simulink model "SRM_IOT"  (R2024b)
settings: Solver=VariableStepAuto  StartTime=0.0  StopTime=10.0  RelTol=1e-3
undefined symbols (not defined in the file): Ion, Lithium, sigbuilder_block
libraries: spsBreakerLib x120, spsSeriesRLCBranchLib x70, spsBatteryLib x42, spsIdealSwitchLib x33, spsVoltageMeasurementLib x27, slpidlib x17, spsMosfetLib x17, spsPWMGeneratorDCDCLib x11, spsDiodeLib x6, spsCurrentMeasurementLib x4, spsIGBTLib x2, spsThreePhaseSeriesRLCLoadLib x2
(part 4 of 5)

== system SRM_IOT/Grid/Wall charger Connection Box/DC-AC // AC-DC Converter ==
  Controller : Subsystem
  Measurement1 : spsThreePhaseVIMeasurementLib/Three-Phase V-I Measurement  VoltageMeasurement=phase-to-ground  SetLabelV=on  LabelV=Vabc_inv  Vpu=off  VpuLL=off  CurrentMeasurement=yes  SetLabelI=on  LabelI=Iabc_inv  Ipu=off  Pbase=100e6  Vbase=500e3  OutputType=Complex  PhasorSimulation=off  PSBequivalent=0
  PWM Generator (2-Level) : spsPWMGenerator2LevelLib/PWM Generator (2-Level)  ModulatorType=Three-phase bridge (6 pulses)  ModulatorMode=Unsynchronized  Fc=4950  Pc=90  nF=27  MinMax="[ -1  1 ]"  SamplingTechnique=Natural  ModulatingSignals=off  m=0.8  Freq=60  Phase=0  Ts=2.02e-6  ShowCarrierOutport=off
  Parallel Connection control : Constant
  Series RLC Branch2 : spsSeriesRLCBranchLib/Series RLC Branch  LConnTagsString=__new0  RConnTagsString=__new0  BranchType=RC  Resistance=10e3  Inductance=1e-3  SetiL0=off  InitialCurrent=0  Capacitance=1000e-6  Setx0=off  InitialVoltage=0  Measurements=None
  Three-Phase Series RLC Branch : spsThreePhaseSeriesRLCBranchLib/Three-Phase Series RLC Branch  LConnTagsString=A|B|C  RConnTagsString=A|B|C  BranchType=RL  Resistance=0.004332  Inductance=0.0013789184  Capacitance=1e-6  Measurements=None
  Three-Phase Breaker : spsThreePhaseBreakerLib/Three-Phase Breaker  InitialState=open  SwitchA=on  SwitchB=on  SwitchC=on  SwitchTimes="[1/60  5/60]"  External=on  BreakerResistance=0.01  SnubberResistance=1e6  SnubberCapacitance=inf  Measurements=None
  Transformer near home1 : spsThreePhaseSeriesRLCLoadLib/Three-Phase Series RLC Load  LConnTagsString=A|B|C  Configuration=Delta  NominalVoltage=380  Vabc=[1e3 1e3 1e3]  Vabcp=[1e3 1e3 1e3]  NominalFrequency=50  UnbalancedPower=off  ActivePower=100  InductivePower=0  CapacitivePower=5000  Pabc=[10e3 9e3 11e3]  QLabc=[100 90 110]  QCabc=[100 90 110]  Pabcp=[10e3 9e3 11e3]  QLabcp=[100 90 110]  QCabcp=[100 90 110]  Measurements=None  LoadType=constant Z
  Universal Bridge : spsUniversalBridgeLib/Universal Bridge  Arms=3  SnubberResistance=1e5  SnubberCapacitance=inf  Device=IGBT / Diodes  Ron=1e-3  Lon=0  ForwardVoltages="[  0  0  ]"  ForwardVoltage=0  GTOparameters=[ 10e-6 , 20e-6 ]  IGBTparameters=[ 1e-6 , 2e-6 ]  Measurements=None  Measurements_2=None  converterType=Rectifier
  Universal Bridge1 : spsUniversalBridgeLib/Universal Bridge  Arms=3  SnubberResistance=1e5  SnubberCapacitance=inf  Device=Diodes  Ron=1e-3  Lon=0  ForwardVoltages="[  0  0  ]"  ForwardVoltage=0  GTOparameters=[ 10e-6 , 20e-6 ]  IGBTparameters=[ 1e-6 , 2e-6 ]  Measurements=None  Measurements_2=None  converterType=Rectifier
  Discharge_R : PMIOPort  Side=Left
  Discharge_Y : PMIOPort  Port=2  Side=Left
  Discharge_B : PMIOPort  Port=3  Side=Left
  charge_R : PMIOPort  Port=4  Side=Left
  charge_Y : PMIOPort  Port=5  Side=Left
  charge_B : PMIOPort  Port=6  Side=Left
  Discharge + : PMIOPort  Port=7  Side=Right
  Discharge - : PMIOPort  Port=8  Side=Right
  charge+ : PMIOPort  Port=9  Side=Right
  charge- : PMIOPort  Port=10  Side=Right
  wires:
  PWM Generator (2-Level)/1 -> Universal Bridge/1
  Parallel Connection control/1 -> Three-Phase Breaker/1
  [ref] -> PWM Generator (2-Level)/1
  connections:
  Universal Bridge1/LConn2 -- charge_Y/RConn1
  Universal Bridge1/LConn3 -- charge_B/RConn1
  Discharge_Y/RConn1 -- Three-Phase Breaker/RConn2
  Three-Phase Series RLC Branch/RConn1 -- Transformer near home1/LConn1 -- Measurement1/LConn1
  Measurement1/RConn2 -- Three-Phase Breaker/LConn2
  charge-/RConn1 -- Series RLC Branch2/RConn1 -- Universal Bridge1/RConn2
  Three-Phase Series RLC Branch/RConn3 -- Measurement1/LConn3 -- Transformer near home1/LConn3
  Discharge_B/RConn1 -- Three-Phase Breaker/RConn3
  Three-Phase Series RLC Branch/LConn2 -- Universal Bridge/LConn2
  Universal Bridge/LConn1 -- Three-Phase Series RLC Branch/LConn1
  Discharge -/RConn1 -- Universal Bridge/RConn2
  Universal Bridge/LConn3 -- Three-Phase Series RLC Branch/LConn3
  Three-Phase Series RLC Branch/RConn2 -- Measurement1/LConn2 -- Transformer near home1/LConn2
  Discharge +/RConn1 -- Universal Bridge/RConn1
  charge+/RConn1 -- Series RLC Branch2/LConn1 -- Universal Bridge1/RConn1
  Discharge_R/RConn1 -- Three-Phase Breaker/RConn1
  Measurement1/RConn1 -- Three-Phase Breaker/LConn1
  Measurement1/RConn3 -- Three-Phase Breaker/LConn3
  Universal Bridge1/LConn1 -- charge_R/RConn1

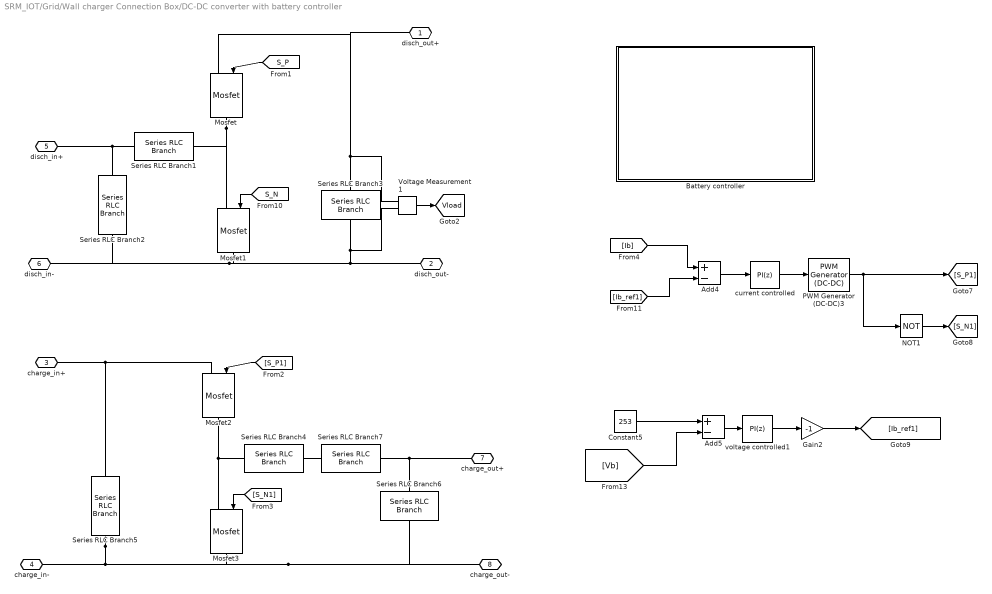
== system SRM_IOT/Grid/Wall charger Connection Box/DC-DC converter with battery controller ==
  Add4 : Sum  Inputs=+-
  Add5 : Sum  Inputs=+-
  Battery controller : Subsystem
  Constant5 : Constant  Value=253
  Gain2 : Gain  Gain=-1
  Mosfet{,1..3} (4 alike) : spsMosfetLib/Mosfet  Ron=0.1  Lon=0  Rd=0.01  Vfd=0  IC=0  Rs=1e5  Cs=inf  Measurements=off
  NOT1 : Logic  Operator=NOT  IconShape=distinctive  AllPortsSameDT=off  OutDataTypeStr=boolean
  PWM Generator (DC-DC)3 : spsPWMGeneratorDCDCLib/PWM Generator (DC-DC)  Fsw=10e3  Ts=5e-6
  Series RLC Branch1 : spsSeriesRLCBranchLib/Series RLC Branch  LConnTagsString=__new0  RConnTagsString=__new0  BranchType=RL  Resistance=1000  Inductance=5.76e-4  SetiL0=off  InitialCurrent=0  Capacitance=1e-6  Setx0=off  InitialVoltage=0  Measurements=None
  Series RLC Branch2 : spsSeriesRLCBranchLib/Series RLC Branch  LConnTagsString=__new0  RConnTagsString=__new0  BranchType=R  Resistance=10  Inductance=1e-3  SetiL0=off  InitialCurrent=0  Capacitance=1000e-6  Setx0=off  InitialVoltage=0  Measurements=None
  Series RLC Branch3 : spsSeriesRLCBranchLib/Series RLC Branch  LConnTagsString=__new0  RConnTagsString=__new0  BranchType=RC  Resistance=0.001  Inductance=1e-3  SetiL0=off  InitialCurrent=0  Capacitance=1000e-6  Setx0=off  InitialVoltage=0  Measurements=None
  Series RLC Branch4 : spsSeriesRLCBranchLib/Series RLC Branch  LConnTagsString=__new0  RConnTagsString=__new0  BranchType=RL  Resistance=0.05  Inductance=5.76e-4  SetiL0=off  InitialCurrent=0  Capacitance=1000e-6  Setx0=off  InitialVoltage=0  Measurements=None
  Series RLC Branch5 : spsSeriesRLCBranchLib/Series RLC Branch  LConnTagsString=__new0  RConnTagsString=__new0  BranchType=RC  Resistance=0.001  Inductance=1e-3  SetiL0=off  InitialCurrent=0  Capacitance=1000e-6  Setx0=off  InitialVoltage=0  Measurements=None
  Series RLC Branch6 : spsSeriesRLCBranchLib/Series RLC Branch  LConnTagsString=__new0  RConnTagsString=__new0  BranchType=RC  Resistance=1e-3  Inductance=1e-3  SetiL0=off  InitialCurrent=0  Capacitance=5600e-6  Setx0=off  InitialVoltage=0  Measurements=None
  Series RLC Branch7 : spsSeriesRLCBranchLib/Series RLC Branch  LConnTagsString=__new0  RConnTagsString=__new0  BranchType=R  Resistance=10  Inductance=1e-3  SetiL0=off  InitialCurrent=0  Capacitance=1000e-6  Setx0=off  InitialVoltage=0  Measurements=None
  Voltage Measurement1 : spsVoltageMeasurementLib/Voltage Measurement  PhasorSimulation=off  OutputType=Complex  PSBequivalent=0
  current controlled : slpidlib/PID Controller  Controller=PI  Form=Parallel  TimeDomain=Discrete-time  UseExternalTs=off  SampleTime=500e-6  IntegratorMethod=Forward Euler  FilterMethod=Forward Euler  ControllerParametersSource=internal  P=0.005  I=10  UseKiTs=off  D=0  UseExternalDerivativeSource=off  N=100  UseFilter=on  TunerSelectOption=Transfer Function Based (PID Tuner App)  InitialConditionSource=internal  InitialConditionForIntegrator=0.54  InitialConditionForFilter=0  DifferentiatorICPrevScaledInput=0  ExternalReset=none  TrackingMode=off  Kt=1  LimitOutput=on  SatLimitsSource=internal  UpperSaturationLimit=0.95  LowerSaturationLimit=0  LinearizeAsGain=on  AntiWindupMode=none  Kb=1  LimitIntegrator=off  UpperIntegratorSaturationLimit=inf  LowerIntegratorSaturationLimit=-inf  POutMin=[]  POutMax=[]  IOutMin=[]  IOutMax=[]  DOutMin=[]  DOutMax=[]  NOutMin=[]  NOutMax=[]  SumOutMin=[]  SumOutMax=[]  SaturationOutMin=[]  SaturationOutMax=[]  PParamMin=[]  PParamMax=[]  IParamMin=[]  IParamMax=[]  DParamMin=[]  DParamMax=[]  NParamMin=[]  NParamMax=[]  KbParamMin=[]  KbParamMax=[]  KtParamMin=[]  KtParamMax=[]  KbOutMin=[]  KbOutMax=[]  KtOutMin=[]  KtOutMax=[]  IntegratorOutMin=[]  IntegratorOutMax=[]  FilterOutMin=[]  FilterOutMax=[]  SumI1OutMin=[]  SumI1OutMax=[]  SumI2OutMin=[]  SumI2OutMax=[]  SumI3OutMin=[]  SumI3OutMax=[]  SumI4OutMin=[]  SumI4OutMax=[]  SumDOutMin=[]  SumDOutMax=[]  DifferentiatorOutMin=[]  DifferentiatorOutMax=[]  FilterDiffOutCoefMin=[]  FilterDiffOutCoefMax=[]  ReciprocalOutMin=[]  ReciprocalOutMax=[]  SumDenOutMin=[]  SumDenOutMax=[]  SumNumOutMin=[]  SumNumOutMax=[]  DivideOutMin=[]  DivideOutMax=[]  UdiffTsProdOutMin=[]  UdiffTsProdOutMax=[]  NTsProdOutMin=[]  NTsProdOutMax=[]  UintegralTsProdOutMin=[]  UintegralTsProdOutMax=[]  UngainTsProdOutMin=[]  UngainTsProdOutMax=[]  ClampingZeroOutDataTypeStr=Inherit: Inherit via back propagation  ClampingZeroOutMin=[]  ClampingZeroOutMax=[]  FilterDenConstantOutDataTypeStr=Inherit: Inherit via back propagation  FilterDenConstantOutMin=[]  FilterDenConstantOutMax=[]  PCopyOutDataTypeStr=Inherit: Inherit via back propagation  PCopyOutMin=[]  PCopyOutMax=[]  NCopyOutDataTypeStr=Inherit: Inherit via back propagation  NCopyOutMin=[]  NCopyOutMax=[]  IntegratorContinuousStateAttributes=''  IntegratorStateMustResolveToSignalObject=off  IntegratorRTWStateStorageClass=Auto  FilterContinuousStateAttributes=''  FilterStateMustResolveToSignalObject=off  FilterRTWStateStorageClass=Auto  ParallelPVariant=InternalParameters  IdealPVariant=Disabled  IVariant=InternalParameters  DVariant=Disabled  IntegratorVariant=Discrete  SatVariant=Enabled  AWVariant=Passthrough  PCopyVariant=Disabled  TRVariant=Disabled  FdbkBlocksVariant=Forward  IdealPFdbkVariant=Disabled  SatFdbkVariant=Disabled  DerivativeFilterVariant=Disabled  NVariant=Disabled  NCopyVariant=Disabled_SignalSpec  FilterICVariant=Disabled  IntegratorICVariant=InternalICs  ExternalResetVariant=Disabled  TRSumVariant=Passthrough  SumFdbkVariant=Disabled  SumVariant=Sum_PI  TsampFilterVariant=InternalTs  TsampNgainVariant=Passthrough  TsampIntegralVariant=Disabled_SignalSpec  ExternalSaturationOutDataTypeStr=Inherit: Same as second input  DerivativeSourceVariant=Disabled  PreIntVariant=InternalPreInt
  voltage controlled1 : slpidlib/PID Controller  Controller=PI  Form=Parallel  TimeDomain=Discrete-time  UseExternalTs=off  SampleTime=500e-6  IntegratorMethod=Forward Euler  FilterMethod=Forward Euler  ControllerParametersSource=internal  P=40  I=2000  UseKiTs=off  D=0  UseExternalDerivativeSource=off  N=100  UseFilter=on  TunerSelectOption=Transfer Function Based (PID Tuner App)  InitialConditionSource=internal  InitialConditionForIntegrator=0  InitialConditionForFilter=0  DifferentiatorICPrevScaledInput=0  ExternalReset=none  TrackingMode=off  Kt=1  LimitOutput=on  SatLimitsSource=internal  UpperSaturationLimit=22  LowerSaturationLimit=0  LinearizeAsGain=on  AntiWindupMode=none  Kb=1  LimitIntegrator=off  UpperIntegratorSaturationLimit=inf  LowerIntegratorSaturationLimit=-inf  POutMin=[]  POutMax=[]  IOutMin=[]  IOutMax=[]  DOutMin=[]  DOutMax=[]  NOutMin=[]  NOutMax=[]  SumOutMin=[]  SumOutMax=[]  SaturationOutMin=[]  SaturationOutMax=[]  PParamMin=[]  PParamMax=[]  IParamMin=[]  IParamMax=[]  DParamMin=[]  DParamMax=[]  NParamMin=[]  NParamMax=[]  KbParamMin=[]  KbParamMax=[]  KtParamMin=[]  KtParamMax=[]  KbOutMin=[]  KbOutMax=[]  KtOutMin=[]  KtOutMax=[]  IntegratorOutMin=[]  IntegratorOutMax=[]  FilterOutMin=[]  FilterOutMax=[]  SumI1OutMin=[]  SumI1OutMax=[]  SumI2OutMin=[]  SumI2OutMax=[]  SumI3OutMin=[]  SumI3OutMax=[]  SumI4OutMin=[]  SumI4OutMax=[]  SumDOutMin=[]  SumDOutMax=[]  DifferentiatorOutMin=[]  DifferentiatorOutMax=[]  FilterDiffOutCoefMin=[]  FilterDiffOutCoefMax=[]  ReciprocalOutMin=[]  ReciprocalOutMax=[]  SumDenOutMin=[]  SumDenOutMax=[]  SumNumOutMin=[]  SumNumOutMax=[]  DivideOutMin=[]  DivideOutMax=[]  UdiffTsProdOutMin=[]  UdiffTsProdOutMax=[]  NTsProdOutMin=[]  NTsProdOutMax=[]  UintegralTsProdOutMin=[]  UintegralTsProdOutMax=[]  UngainTsProdOutMin=[]  UngainTsProdOutMax=[]  ClampingZeroOutDataTypeStr=Inherit: Inherit via back propagation  ClampingZeroOutMin=[]  ClampingZeroOutMax=[]  FilterDenConstantOutDataTypeStr=Inherit: Inherit via back propagation  FilterDenConstantOutMin=[]  FilterDenConstantOutMax=[]  PCopyOutDataTypeStr=Inherit: Inherit via back propagation  PCopyOutMin=[]  PCopyOutMax=[]  NCopyOutDataTypeStr=Inherit: Inherit via back propagation  NCopyOutMin=[]  NCopyOutMax=[]  IntegratorContinuousStateAttributes=''  IntegratorStateMustResolveToSignalObject=off  IntegratorRTWStateStorageClass=Auto  FilterContinuousStateAttributes=''  FilterStateMustResolveToSignalObject=off  FilterRTWStateStorageClass=Auto  ParallelPVariant=InternalParameters  IdealPVariant=Disabled  IVariant=InternalParameters  DVariant=Disabled  IntegratorVariant=Discrete  SatVariant=Enabled  AWVariant=Passthrough  PCopyVariant=Disabled  TRVariant=Disabled  FdbkBlocksVariant=Forward  IdealPFdbkVariant=Disabled  SatFdbkVariant=Disabled  DerivativeFilterVariant=Disabled  NVariant=Disabled  NCopyVariant=Disabled_SignalSpec  FilterICVariant=Disabled  IntegratorICVariant=InternalICs  ExternalResetVariant=Disabled  TRSumVariant=Passthrough  SumFdbkVariant=Disabled  SumVariant=Sum_PI  TsampFilterVariant=InternalTs  TsampNgainVariant=Passthrough  TsampIntegralVariant=Disabled_SignalSpec  ExternalSaturationOutDataTypeStr=Inherit: Same as second input  DerivativeSourceVariant=Disabled  PreIntVariant=InternalPreInt
  disch_out+ : PMIOPort  Side=Left
  disch_out- : PMIOPort  Port=2  Side=Left
  charge_in+ : PMIOPort  Port=3  Side=Left
  charge_in- : PMIOPort  Port=4  Side=Left
  disch_in+ : PMIOPort  Port=5  Side=Right
  disch_in- : PMIOPort  Port=6  Side=Right
  charge_out+ : PMIOPort  Port=7  Side=Right
  charge_out- : PMIOPort  Port=8  Side=Right
  tag scope: Vload=global
  wires:
  [S_P1] -> Mosfet2/1
  Add5/1 -> voltage controlled1/1
  [S_N1] -> Mosfet3/1
  PWM Generator (DC-DC)3/1 -> NOT1/1, [S_P1]
  Gain2/1 -> [Ib_ref1]
  [S_N] -> Mosfet1/1
  [S_P] -> Mosfet/1
  Constant5/1 -> Add5/1
  Voltage Measurement1/1 -> [Vload]
  [Ib_ref1] -> Add4/2
  voltage controlled1/1 -> Gain2/1
  current controlled/1 -> PWM Generator (DC-DC)3/1
  Add4/1 -> current controlled/1
  NOT1/1 -> [S_N1]
  [Vb] -> Add5/2
  [Ib] -> Add4/1
  connections:
  Series RLC Branch5/RConn1 -- charge_in-/RConn1 -- Mosfet3/RConn1 -- charge_out-/RConn1 -- Series RLC Branch6/RConn1
  Mosfet3/LConn1 -- Mosfet2/RConn1 -- Series RLC Branch4/LConn1
  Series RLC Branch5/LConn1 -- charge_in+/RConn1 -- Mosfet2/LConn1
  Series RLC Branch3/LConn1 -- disch_out+/RConn1 -- Mosfet/LConn1 -- Voltage Measurement1/LConn1
  Series RLC Branch6/LConn1 -- charge_out+/RConn1 -- Series RLC Branch7/LConn1
  Series RLC Branch3/RConn1 -- Voltage Measurement1/LConn2 -- disch_out-/RConn1 -- Mosfet1/RConn1 -- disch_in-/RConn1 -- Series RLC Branch2/RConn1
  Series RLC Branch4/RConn1 -- Series RLC Branch7/RConn1
  Mosfet/RConn1 -- Series RLC Branch1/RConn1 -- Mosfet1/LConn1
  Series RLC Branch2/LConn1 -- disch_in+/RConn1 -- Series RLC Branch1/LConn1

== system SRM_IOT/MPPT and PV Controller/Inverter controller/Inverter Controller ==
  V_Dc : Inport
  370 : Inport  Port=2
  V_Sys_Secondary : Inport  Port=3
  I_Sys_Secondary : Inport  Port=4
  Enable : EnablePort  StatesWhenEnabling=reset
  Add : Sum
  Add1 : Sum  Inputs=+-|
  Add2 : Sum  Inputs=+-|
  Constant : Constant  Value=-1
  Constant4 : Constant
  Divide1 : Product  Inputs=*/
  Gain : Gain  Gain=2
  PLL : spsPLLLib/PLL  Fmin=45  Par_Init=[0, 60]  ParK=[180, 3200, 1]  TcD=1e-4  MaxRateChangeFreq=12  FilterCutOffFreq=25  Ts=0  AGC=on
  PWM Generator (2-Level) : spsPWMGenerator2LevelLib/PWM Generator (2-Level)  ModulatorType=Single-phase full-bridge (4 pulses)  ModulatorMode=Unsynchronized  Fc=10000  Pc=90  nF=27  MinMax="[ -1  1 ]"  SamplingTechnique=Natural  ModulatingSignals=off  m=0.8  Freq=60  Phase=0  Ts=0  ShowCarrierOutport=off
  Product1 : Product  RndMeth=Zero
  Saturation1 : Saturate  UpperLimit=1  LowerLimit=-1
  Saturation3 : Saturate  UpperLimit=50  LowerLimit=-50
  Terminator : Terminator
  Transfer Fcn1 : TransferFcn  Denominator=[1e-4 1]
  Transfer Fcn2 : TransferFcn  Denominator=[1e-4 1]
  Transfer Fcn3 : TransferFcn  Denominator=[1e-4 1]
  Trigonometric Function : Trigonometry
  Pulse : Outport  OutputWhenDisabled=reset  InitialOutput=[0 0 0 0]  VectorParamsAs1DForOutWhenUnconnected=off
  wires:
  PWM Generator (2-Level)/1 -> Pulse/1
  370/1 -> Add1/2  "Vref"
  Add/1 -> PWM Generator (2-Level)/1  "duty_to_-1_1"
  Gain/1 -> Add/1
  Constant/1 -> Add/2
  V_Dc/1 -> Add1/1
  Add1/1 -> Transfer Fcn1/1  "err"
  I_Sys_Secondary/1 -> Add2/1
  Add2/1 -> Transfer Fcn2/1  "err"
  Transfer Fcn2/1 -> Saturation1/1  "err_filter"
  Transfer Fcn1/1 -> Saturation3/1  "Iref"
  Product1/1 -> Transfer Fcn3/1
  Saturation1/1 -> Gain/1
  Divide1/1 -> PLL/1  "V_Sys_Secondary"
  PLL/2 -> Trigonometric Function/1  "wt"
  Constant4/1 -> Divide1/2
  V_Sys_Secondary/1 -> Divide1/1
  Transfer Fcn3/1 -> Add2/2
  Saturation3/1 -> Product1/1
  Trigonometric Function/1 -> Product1/2
  PLL/1 -> Terminator/1  "Freq"

== system SRM_IOT/Vechicle BMS Monitoring/BMS Discharge/Function logic block ==
  Terminal voltage : Inport
  Current : Inport  Port=2
  Temperature : Inport  Port=3
  Display : Display
  Display1 : Display
  Display2 : Display
  Max Temp : Constant  Value=333
  Min temp : Constant  Value=253
  OR : Logic  Operator=OR  AllPortsSameDT=off  OutDataTypeStr=boolean
  OR1 : Logic  Operator=OR  Inputs=3  AllPortsSameDT=off  OutDataTypeStr=boolean
  Over current : Constant  Value=155
  Relational Operator : RelationalOperator  Operator=<=  OutDataTypeStr=boolean  RndMeth=Simplest  InputSameDT=off
  Relational Operator1 : RelationalOperator  OutDataTypeStr=boolean  RndMeth=Simplest  InputSameDT=off
  Relational Operator2 : RelationalOperator  OutDataTypeStr=boolean  RndMeth=Simplest  InputSameDT=off
  Relational Operator3 : RelationalOperator  OutDataTypeStr=boolean  RndMeth=Simplest  InputSameDT=off
  Under voltage : Constant  Value=2.7
  Discharge Terget : Outport
  wires:
  Terminal voltage/1 -> Relational Operator/1
  Under voltage/1 -> Relational Operator/2
  Over current/1 -> Relational Operator1/2
  Current/1 -> Relational Operator1/1
  Temperature/1 -> Relational Operator3/1, Relational Operator2/1
  Max Temp/1 -> Relational Operator2/2
  Min temp/1 -> Relational Operator3/2
  Relational Operator2/1 -> OR/1
  Relational Operator3/1 -> OR/2
  OR/1 -> Display2/1, OR1/3
  Relational Operator1/1 -> Display1/1, OR1/2
  Relational Operator/1 -> Display/1, OR1/1
  OR1/1 -> Discharge Terget/1

== system SRM_IOT/Vechicle BMS Monitoring1/BMS Discharge/Function logic block ==
  Terminal voltage : Inport
  Current : Inport  Port=2
  Temperature : Inport  Port=3
  Display : Display
  Display1 : Display
  Display2 : Display
  Max Temp : Constant  Value=333
  Min temp : Constant  Value=253
  OR : Logic  Operator=OR  AllPortsSameDT=off  OutDataTypeStr=boolean
  OR1 : Logic  Operator=OR  Inputs=3  AllPortsSameDT=off  OutDataTypeStr=boolean
  Over current : Constant  Value=155
  Relational Operator : RelationalOperator  Operator=<=  OutDataTypeStr=boolean  RndMeth=Simplest  InputSameDT=off
  Relational Operator1 : RelationalOperator  OutDataTypeStr=boolean  RndMeth=Simplest  InputSameDT=off
  Relational Operator2 : RelationalOperator  OutDataTypeStr=boolean  RndMeth=Simplest  InputSameDT=off
  Relational Operator3 : RelationalOperator  OutDataTypeStr=boolean  RndMeth=Simplest  InputSameDT=off
  Under voltage : Constant  Value=2.7
  Discharge Terget : Outport
  wires:
  Terminal voltage/1 -> Relational Operator/1
  Under voltage/1 -> Relational Operator/2
  Over current/1 -> Relational Operator1/2
  Current/1 -> Relational Operator1/1
  Temperature/1 -> Relational Operator3/1, Relational Operator2/1
  Max Temp/1 -> Relational Operator2/2
  Min temp/1 -> Relational Operator3/2
  Relational Operator2/1 -> OR/1
  Relational Operator3/1 -> OR/2
  OR/1 -> Display2/1, OR1/3
  Relational Operator1/1 -> Display1/1, OR1/2
  Relational Operator/1 -> Display/1, OR1/1
  OR1/1 -> Discharge Terget/1

== system SRM_IOT/Vechicle BMS Monitoring2/BMS Discharge/Function logic block ==
  Terminal voltage : Inport
  Current : Inport  Port=2
  Temperature : Inport  Port=3
  Display : Display
  Display1 : Display
  Display2 : Display
  Max Temp : Constant  Value=333
  Min temp : Constant  Value=253
  OR : Logic  Operator=OR  AllPortsSameDT=off  OutDataTypeStr=boolean
  OR1 : Logic  Operator=OR  Inputs=3  AllPortsSameDT=off  OutDataTypeStr=boolean
  Over current : Constant  Value=155
  Relational Operator : RelationalOperator  Operator=<=  OutDataTypeStr=boolean  RndMeth=Simplest  InputSameDT=off
  Relational Operator1 : RelationalOperator  OutDataTypeStr=boolean  RndMeth=Simplest  InputSameDT=off
  Relational Operator2 : RelationalOperator  OutDataTypeStr=boolean  RndMeth=Simplest  InputSameDT=off
  Relational Operator3 : RelationalOperator  OutDataTypeStr=boolean  RndMeth=Simplest  InputSameDT=off
  Under voltage : Constant  Value=2.7
  Discharge Terget : Outport
  wires:
  Terminal voltage/1 -> Relational Operator/1
  Under voltage/1 -> Relational Operator/2
  Over current/1 -> Relational Operator1/2
  Current/1 -> Relational Operator1/1
  Temperature/1 -> Relational Operator3/1, Relational Operator2/1
  Max Temp/1 -> Relational Operator2/2
  Min temp/1 -> Relational Operator3/2
  Relational Operator2/1 -> OR/1
  Relational Operator3/1 -> OR/2
  OR/1 -> Display2/1, OR1/3
  Relational Operator1/1 -> Display1/1, OR1/2
  Relational Operator/1 -> Display/1, OR1/1
  OR1/1 -> Discharge Terget/1

== system SRM_IOT/Vechicle BMS Monitoring3/BMS Discharge/Function logic block ==
  Terminal voltage : Inport
  Current : Inport  Port=2
  Temperature : Inport  Port=3
  Display : Display
  Display1 : Display
  Display2 : Display
  Max Temp : Constant  Value=333
  Min temp : Constant  Value=253
  OR : Logic  Operator=OR  AllPortsSameDT=off  OutDataTypeStr=boolean
  OR1 : Logic  Operator=OR  Inputs=3  AllPortsSameDT=off  OutDataTypeStr=boolean
  Over current : Constant  Value=155
  Relational Operator : RelationalOperator  Operator=<=  OutDataTypeStr=boolean  RndMeth=Simplest  InputSameDT=off
  Relational Operator1 : RelationalOperator  OutDataTypeStr=boolean  RndMeth=Simplest  InputSameDT=off
  Relational Operator2 : RelationalOperator  OutDataTypeStr=boolean  RndMeth=Simplest  InputSameDT=off
  Relational Operator3 : RelationalOperator  OutDataTypeStr=boolean  RndMeth=Simplest  InputSameDT=off
  Under voltage : Constant  Value=2.7
  Discharge Terget : Outport
  wires:
  Terminal voltage/1 -> Relational Operator/1
  Under voltage/1 -> Relational Operator/2
  Over current/1 -> Relational Operator1/2
  Current/1 -> Relational Operator1/1
  Temperature/1 -> Relational Operator3/1, Relational Operator2/1
  Max Temp/1 -> Relational Operator2/2
  Min temp/1 -> Relational Operator3/2
  Relational Operator2/1 -> OR/1
  Relational Operator3/1 -> OR/2
  OR/1 -> Display2/1, OR1/3
  Relational Operator1/1 -> Display1/1, OR1/2
  Relational Operator/1 -> Display/1, OR1/1
  OR1/1 -> Discharge Terget/1

== system SRM_IOT/Grid/Wall charger Connection Box/Buck-Boost Converter/Buck Boost Controller ==
  Add1 : Sum  Inputs=+-
  Add2 : Sum  Inputs=+-
  Constant : Constant  Value=600
  Constant1 : Constant  Value=180
  PID Controller1 : slpidlib/PID Controller  Controller=PID  Form=Parallel  TimeDomain=Continuous-time  UseExternalTs=off  SampleTime=-1  IntegratorMethod=Forward Euler  FilterMethod=Forward Euler  ControllerParametersSource=internal  P=0  I=7  UseKiTs=off  D=0  UseExternalDerivativeSource=off  N=100  UseFilter=on  TunerSelectOption=Transfer Function Based (PID Tuner App)  InitialConditionSource=internal  InitialConditionForIntegrator=0  InitialConditionForFilter=0  DifferentiatorICPrevScaledInput=0  ExternalReset=none  TrackingMode=off  Kt=1  LimitOutput=off  SatLimitsSource=internal  UpperSaturationLimit=inf  LowerSaturationLimit=-inf  LinearizeAsGain=on  AntiWindupMode=none  Kb=1  LimitIntegrator=off  UpperIntegratorSaturationLimit=inf  LowerIntegratorSaturationLimit=-inf  POutMin=[]  POutMax=[]  IOutMin=[]  IOutMax=[]  DOutMin=[]  DOutMax=[]  NOutMin=[]  NOutMax=[]  SumOutMin=[]  SumOutMax=[]  SaturationOutMin=[]  SaturationOutMax=[]  PParamMin=[]  PParamMax=[]  IParamMin=[]  IParamMax=[]  DParamMin=[]  DParamMax=[]  NParamMin=[]  NParamMax=[]  KbParamMin=[]  KbParamMax=[]  KtParamMin=[]  KtParamMax=[]  KbOutMin=[]  KbOutMax=[]  KtOutMin=[]  KtOutMax=[]  IntegratorOutMin=[]  IntegratorOutMax=[]  FilterOutMin=[]  FilterOutMax=[]  SumI1OutMin=[]  SumI1OutMax=[]  SumI2OutMin=[]  SumI2OutMax=[]  SumI3OutMin=[]  SumI3OutMax=[]  SumI4OutMin=[]  SumI4OutMax=[]  SumDOutMin=[]  SumDOutMax=[]  DifferentiatorOutMin=[]  DifferentiatorOutMax=[]  FilterDiffOutCoefMin=[]  FilterDiffOutCoefMax=[]  ReciprocalOutMin=[]  ReciprocalOutMax=[]  SumDenOutMin=[]  SumDenOutMax=[]  SumNumOutMin=[]  SumNumOutMax=[]  DivideOutMin=[]  DivideOutMax=[]  UdiffTsProdOutMin=[]  UdiffTsProdOutMax=[]  NTsProdOutMin=[]  NTsProdOutMax=[]  UintegralTsProdOutMin=[]  UintegralTsProdOutMax=[]  UngainTsProdOutMin=[]  UngainTsProdOutMax=[]  ClampingZeroOutDataTypeStr=Inherit: Inherit via back propagation  ClampingZeroOutMin=[]  ClampingZeroOutMax=[]  FilterDenConstantOutDataTypeStr=Inherit: Inherit via back propagation  FilterDenConstantOutMin=[]  FilterDenConstantOutMax=[]  PCopyOutDataTypeStr=Inherit: Inherit via back propagation  PCopyOutMin=[]  PCopyOutMax=[]  NCopyOutDataTypeStr=Inherit: Inherit via back propagation  NCopyOutMin=[]  NCopyOutMax=[]  IntegratorContinuousStateAttributes=''  IntegratorStateMustResolveToSignalObject=off  IntegratorRTWStateStorageClass=Auto  FilterContinuousStateAttributes=''  FilterStateMustResolveToSignalObject=off  FilterRTWStateStorageClass=Auto  ParallelPVariant=InternalParameters  IdealPVariant=Disabled  IVariant=InternalParameters  DVariant=InternalParameters  IntegratorVariant=Continuous  SatVariant=Disabled  AWVariant=Passthrough  PCopyVariant=Disabled  TRVariant=Disabled  FdbkBlocksVariant=Forward  IdealPFdbkVariant=Disabled  SatFdbkVariant=Disabled  DerivativeFilterVariant=ContFilter  NVariant=InternalParameters  NCopyVariant=Disabled  FilterICVariant=InternalICsFilter  IntegratorICVariant=InternalICs  ExternalResetVariant=Disabled  TRSumVariant=Passthrough  SumFdbkVariant=Disabled  SumVariant=Sum_PID  TsampFilterVariant=InternalTs  TsampNgainVariant=Passthrough  TsampIntegralVariant=Disabled_SignalSpec  ExternalSaturationOutDataTypeStr=Inherit: Same as second input  DerivativeSourceVariant=ErrorSignal  PreIntVariant=InternalPreInt
  PID Controller2 : slpidlib/PID Controller  Controller=PID  Form=Parallel  TimeDomain=Continuous-time  UseExternalTs=off  SampleTime=-1  IntegratorMethod=Forward Euler  FilterMethod=Forward Euler  ControllerParametersSource=internal  P=0  I=7  UseKiTs=off  D=0  UseExternalDerivativeSource=off  N=100  UseFilter=on  TunerSelectOption=Transfer Function Based (PID Tuner App)  InitialConditionSource=internal  InitialConditionForIntegrator=0  InitialConditionForFilter=0  DifferentiatorICPrevScaledInput=0  ExternalReset=none  TrackingMode=off  Kt=1  LimitOutput=off  SatLimitsSource=internal  UpperSaturationLimit=inf  LowerSaturationLimit=-inf  LinearizeAsGain=on  AntiWindupMode=none  Kb=1  LimitIntegrator=off  UpperIntegratorSaturationLimit=inf  LowerIntegratorSaturationLimit=-inf  POutMin=[]  POutMax=[]  IOutMin=[]  IOutMax=[]  DOutMin=[]  DOutMax=[]  NOutMin=[]  NOutMax=[]  SumOutMin=[]  SumOutMax=[]  SaturationOutMin=[]  SaturationOutMax=[]  PParamMin=[]  PParamMax=[]  IParamMin=[]  IParamMax=[]  DParamMin=[]  DParamMax=[]  NParamMin=[]  NParamMax=[]  KbParamMin=[]  KbParamMax=[]  KtParamMin=[]  KtParamMax=[]  KbOutMin=[]  KbOutMax=[]  KtOutMin=[]  KtOutMax=[]  IntegratorOutMin=[]  IntegratorOutMax=[]  FilterOutMin=[]  FilterOutMax=[]  SumI1OutMin=[]  SumI1OutMax=[]  SumI2OutMin=[]  SumI2OutMax=[]  SumI3OutMin=[]  SumI3OutMax=[]  SumI4OutMin=[]  SumI4OutMax=[]  SumDOutMin=[]  SumDOutMax=[]  DifferentiatorOutMin=[]  DifferentiatorOutMax=[]  FilterDiffOutCoefMin=[]  FilterDiffOutCoefMax=[]  ReciprocalOutMin=[]  ReciprocalOutMax=[]  SumDenOutMin=[]  SumDenOutMax=[]  SumNumOutMin=[]  SumNumOutMax=[]  DivideOutMin=[]  DivideOutMax=[]  UdiffTsProdOutMin=[]  UdiffTsProdOutMax=[]  NTsProdOutMin=[]  NTsProdOutMax=[]  UintegralTsProdOutMin=[]  UintegralTsProdOutMax=[]  UngainTsProdOutMin=[]  UngainTsProdOutMax=[]  ClampingZeroOutDataTypeStr=Inherit: Inherit via back propagation  ClampingZeroOutMin=[]  ClampingZeroOutMax=[]  FilterDenConstantOutDataTypeStr=Inherit: Inherit via back propagation  FilterDenConstantOutMin=[]  FilterDenConstantOutMax=[]  PCopyOutDataTypeStr=Inherit: Inherit via back propagation  PCopyOutMin=[]  PCopyOutMax=[]  NCopyOutDataTypeStr=Inherit: Inherit via back propagation  NCopyOutMin=[]  NCopyOutMax=[]  IntegratorContinuousStateAttributes=''  IntegratorStateMustResolveToSignalObject=off  IntegratorRTWStateStorageClass=Auto  FilterContinuousStateAttributes=''  FilterStateMustResolveToSignalObject=off  FilterRTWStateStorageClass=Auto  ParallelPVariant=InternalParameters  IdealPVariant=Disabled  IVariant=InternalParameters  DVariant=InternalParameters  IntegratorVariant=Continuous  SatVariant=Disabled  AWVariant=Passthrough  PCopyVariant=Disabled  TRVariant=Disabled  FdbkBlocksVariant=Forward  IdealPFdbkVariant=Disabled  SatFdbkVariant=Disabled  DerivativeFilterVariant=ContFilter  NVariant=InternalParameters  NCopyVariant=Disabled  FilterICVariant=InternalICsFilter  IntegratorICVariant=InternalICs  ExternalResetVariant=Disabled  TRSumVariant=Passthrough  SumFdbkVariant=Disabled  SumVariant=Sum_PID  TsampFilterVariant=InternalTs  TsampNgainVariant=Passthrough  TsampIntegralVariant=Disabled_SignalSpec  ExternalSaturationOutDataTypeStr=Inherit: Same as second input  DerivativeSourceVariant=ErrorSignal  PreIntVariant=InternalPreInt
  PWM Generator (DC-DC) : spsPWMGeneratorDCDCLib/PWM Generator (DC-DC)  Fsw=5000  Ts=0
  PWM Generator (DC-DC)1 : spsPWMGeneratorDCDCLib/PWM Generator (DC-DC)  Fsw=5000  Ts=0
  tag scope: m1=global, m2=global
  wires:
  Constant/1 -> Add1/1
  PID Controller2/1 -> PWM Generator (DC-DC)1/1
  Constant1/1 -> Add2/1
  PWM Generator (DC-DC)1/1 -> [m2]
  [V1] -> Add2/2
  PID Controller1/1 -> PWM Generator (DC-DC)/1
  PWM Generator (DC-DC)/1 -> [m1]
  Add2/1 -> PID Controller2/1
  [V2] -> Add1/2
  Add1/1 -> PID Controller1/1

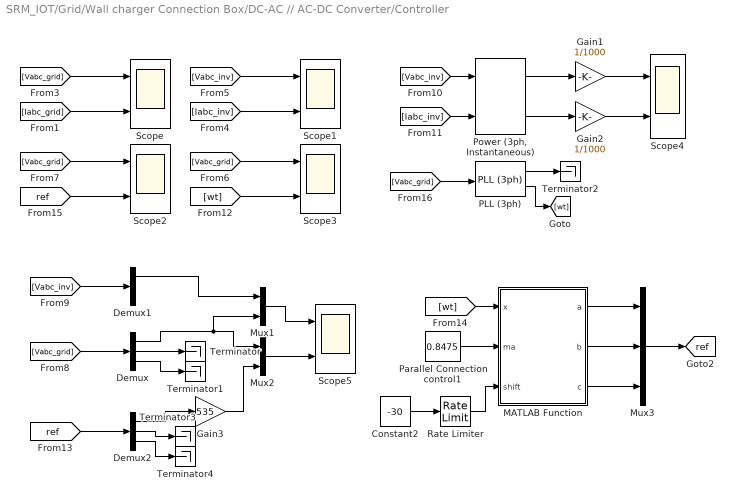
== system SRM_IOT/Grid/Wall charger Connection Box/DC-AC // AC-DC Converter/Controller ==
  Constant2 : Constant  Value=-30
  Demux : Demux  Outputs=3
  Demux1 : Demux  Outputs=3
  Demux2 : Demux  Outputs=3
  Gain1 : Gain  Gain=1/1000
  Gain2 : Gain  Gain=1/1000
  Gain3 : Gain  Gain=535
  MATLAB Function : MATLAB Function  TreatAsAtomicUnit=on
  Mux1 : Mux  Inputs=2
  Mux2 : Mux  Inputs=2
  Mux3 : Mux  Inputs=3
  PLL (3ph) : spsPLL3phLib/PLL (3ph)  Fmin=45  Par_Init=[0, 50]  ParK=[180, 3200, 1]  TcD=1e-4  MaxRateChangeFreq=12  FilterCutOffFreq=25  Ts=0  AGC=on
  Parallel Connection control1 : Constant  Value=0.8475
  "Power (3ph, Instantaneous)" : spsPower3phInstantaneousLib/Power (3ph, Instantaneous)
  Rate Limiter : RateLimiter  SampleTimeMode=inherited
  Scope{,1..5} (6 alike) : Scope  NumInputPorts=2
  Terminator{,1..4} (5 alike) : Terminator
  tag scope: ref=global
  wires:
  Demux1/1 -> Mux1/1
  Mux3/1 -> [ref]
  Gain2/1 -> Scope4/2
  MATLAB Function/2(b) -> Mux3/2
  Gain3/1 -> Mux2/2
  Demux/3 -> Terminator1/1
  [ref] -> Demux2/1
  "Power (3ph, Instantaneous)"/1 -> Gain1/1
  [Iabc_inv] -> "Power (3ph, Instantaneous)"/2
  Constant2/1 -> Rate Limiter/1
  [Vabc_grid] -> PLL (3ph)/1
  Demux2/1 -> Gain3/1
  Demux/2 -> Terminator/1
  PLL (3ph)/1 -> Terminator2/1
  Parallel Connection control1/1 -> MATLAB Function/2(ma)
  "Power (3ph, Instantaneous)"/2 -> Gain2/1
  [ref] -> Scope2/2
  Gain1/1 -> Scope4/1
  [wt] -> MATLAB Function/1(x)
  [Vabc_inv] -> Scope1/1
  Demux2/2 -> Terminator3/1
  MATLAB Function/3(c) -> Mux3/3
  PLL (3ph)/2 -> [wt]
  [wt] -> Scope3/2
  Mux2/1 -> Scope5/2
  [Vabc_grid] -> Scope2/1
  [Iabc_grid] -> Scope/2
  [Iabc_inv] -> Scope1/2
  [Vabc_inv] -> Demux1/1
  Rate Limiter/1 -> MATLAB Function/3(shift)
  Mux1/1 -> Scope5/1
  [Vabc_grid] -> Scope3/1
  [Vabc_inv] -> "Power (3ph, Instantaneous)"/1
  Demux2/3 -> Terminator4/1
  Demux/1 -> Mux1/2, Mux2/1
  [Vabc_grid] -> Scope/1
  MATLAB Function/1(a) -> Mux3/1
  [Vabc_grid] -> Demux/1

== system SRM_IOT/Grid/Wall charger Connection Box/DC-DC converter with battery controller/Battery controller ==
  Add1 : Sum  Inputs=+-
  Add2 : Sum  Inputs=+-
  Add3 : Sum  Inputs=+-
  Constant1 : Constant  Value=48
  Constant2 : Constant  Value=25.98
  Constant4 : Constant
  Current controller : slpidlib/PID Controller  Controller=PI  Form=Parallel  TimeDomain=Discrete-time  UseExternalTs=off  SampleTime=500e-6  IntegratorMethod=Forward Euler  FilterMethod=Forward Euler  ControllerParametersSource=internal  P=0.005  I=10  UseKiTs=off  D=0  UseExternalDerivativeSource=off  N=100  UseFilter=on  TunerSelectOption=Transfer Function Based (PID Tuner App)  InitialConditionSource=internal  InitialConditionForIntegrator=0.54  InitialConditionForFilter=0  DifferentiatorICPrevScaledInput=0  ExternalReset=none  TrackingMode=off  Kt=1  LimitOutput=on  SatLimitsSource=internal  UpperSaturationLimit=0.95  LowerSaturationLimit=0  LinearizeAsGain=on  AntiWindupMode=none  Kb=1  LimitIntegrator=off  UpperIntegratorSaturationLimit=inf  LowerIntegratorSaturationLimit=-inf  POutMin=[]  POutMax=[]  IOutMin=[]  IOutMax=[]  DOutMin=[]  DOutMax=[]  NOutMin=[]  NOutMax=[]  SumOutMin=[]  SumOutMax=[]  SaturationOutMin=[]  SaturationOutMax=[]  PParamMin=[]  PParamMax=[]  IParamMin=[]  IParamMax=[]  DParamMin=[]  DParamMax=[]  NParamMin=[]  NParamMax=[]  KbParamMin=[]  KbParamMax=[]  KtParamMin=[]  KtParamMax=[]  KbOutMin=[]  KbOutMax=[]  KtOutMin=[]  KtOutMax=[]  IntegratorOutMin=[]  IntegratorOutMax=[]  FilterOutMin=[]  FilterOutMax=[]  SumI1OutMin=[]  SumI1OutMax=[]  SumI2OutMin=[]  SumI2OutMax=[]  SumI3OutMin=[]  SumI3OutMax=[]  SumI4OutMin=[]  SumI4OutMax=[]  SumDOutMin=[]  SumDOutMax=[]  DifferentiatorOutMin=[]  DifferentiatorOutMax=[]  FilterDiffOutCoefMin=[]  FilterDiffOutCoefMax=[]  ReciprocalOutMin=[]  ReciprocalOutMax=[]  SumDenOutMin=[]  SumDenOutMax=[]  SumNumOutMin=[]  SumNumOutMax=[]  DivideOutMin=[]  DivideOutMax=[]  UdiffTsProdOutMin=[]  UdiffTsProdOutMax=[]  NTsProdOutMin=[]  NTsProdOutMax=[]  UintegralTsProdOutMin=[]  UintegralTsProdOutMax=[]  UngainTsProdOutMin=[]  UngainTsProdOutMax=[]  ClampingZeroOutDataTypeStr=Inherit: Inherit via back propagation  ClampingZeroOutMin=[]  ClampingZeroOutMax=[]  FilterDenConstantOutDataTypeStr=Inherit: Inherit via back propagation  FilterDenConstantOutMin=[]  FilterDenConstantOutMax=[]  PCopyOutDataTypeStr=Inherit: Inherit via back propagation  PCopyOutMin=[]  PCopyOutMax=[]  NCopyOutDataTypeStr=Inherit: Inherit via back propagation  NCopyOutMin=[]  NCopyOutMax=[]  IntegratorContinuousStateAttributes=''  IntegratorStateMustResolveToSignalObject=off  IntegratorRTWStateStorageClass=Auto  FilterContinuousStateAttributes=''  FilterStateMustResolveToSignalObject=off  FilterRTWStateStorageClass=Auto  ParallelPVariant=InternalParameters  IdealPVariant=Disabled  IVariant=InternalParameters  DVariant=Disabled  IntegratorVariant=Discrete  SatVariant=Enabled  AWVariant=Passthrough  PCopyVariant=Disabled  TRVariant=Disabled  FdbkBlocksVariant=Forward  IdealPFdbkVariant=Disabled  SatFdbkVariant=Disabled  DerivativeFilterVariant=Disabled  NVariant=Disabled  NCopyVariant=Disabled_SignalSpec  FilterICVariant=Disabled  IntegratorICVariant=InternalICs  ExternalResetVariant=Disabled  TRSumVariant=Passthrough  SumFdbkVariant=Disabled  SumVariant=Sum_PI  TsampFilterVariant=InternalTs  TsampNgainVariant=Passthrough  TsampIntegralVariant=Disabled_SignalSpec  ExternalSaturationOutDataTypeStr=Inherit: Same as second input  DerivativeSourceVariant=Disabled  PreIntVariant=InternalPreInt
  Display2 : Display
  Display3 : Display
  Display4 : Display
  Gain1 : Gain  Gain=-1
  NOT1 : Logic  Operator=NOT  IconShape=distinctive  AllPortsSameDT=off  OutDataTypeStr=boolean
  NOT3 : Logic  Operator=NOT  IconShape=distinctive  AllPortsSameDT=off  OutDataTypeStr=boolean
  PWM Generator (DC-DC)1 : spsPWMGeneratorDCDCLib/PWM Generator (DC-DC)  Fsw=10e3  Ts=5e-6
  Switch1 : Switch  Criteria=u2 > Threshold  SaturateOnIntegerOverflow=off  InputSameDT=off
  discharge controlled : slpidlib/PID Controller  Controller=PI  Form=Parallel  TimeDomain=Discrete-time  UseExternalTs=off  SampleTime=500e-6  IntegratorMethod=Forward Euler  FilterMethod=Forward Euler  ControllerParametersSource=internal  P=0.25  I=50  UseKiTs=off  D=0  UseExternalDerivativeSource=off  N=100  UseFilter=on  TunerSelectOption=Transfer Function Based (PID Tuner App)  InitialConditionSource=internal  InitialConditionForIntegrator=0  InitialConditionForFilter=0  DifferentiatorICPrevScaledInput=0  ExternalReset=none  TrackingMode=off  Kt=1  LimitOutput=on  SatLimitsSource=internal  UpperSaturationLimit=22  LowerSaturationLimit=0  LinearizeAsGain=on  AntiWindupMode=none  Kb=1  LimitIntegrator=off  UpperIntegratorSaturationLimit=inf  LowerIntegratorSaturationLimit=-inf  POutMin=[]  POutMax=[]  IOutMin=[]  IOutMax=[]  DOutMin=[]  DOutMax=[]  NOutMin=[]  NOutMax=[]  SumOutMin=[]  SumOutMax=[]  SaturationOutMin=[]  SaturationOutMax=[]  PParamMin=[]  PParamMax=[]  IParamMin=[]  IParamMax=[]  DParamMin=[]  DParamMax=[]  NParamMin=[]  NParamMax=[]  KbParamMin=[]  KbParamMax=[]  KtParamMin=[]  KtParamMax=[]  KbOutMin=[]  KbOutMax=[]  KtOutMin=[]  KtOutMax=[]  IntegratorOutMin=[]  IntegratorOutMax=[]  FilterOutMin=[]  FilterOutMax=[]  SumI1OutMin=[]  SumI1OutMax=[]  SumI2OutMin=[]  SumI2OutMax=[]  SumI3OutMin=[]  SumI3OutMax=[]  SumI4OutMin=[]  SumI4OutMax=[]  SumDOutMin=[]  SumDOutMax=[]  DifferentiatorOutMin=[]  DifferentiatorOutMax=[]  FilterDiffOutCoefMin=[]  FilterDiffOutCoefMax=[]  ReciprocalOutMin=[]  ReciprocalOutMax=[]  SumDenOutMin=[]  SumDenOutMax=[]  SumNumOutMin=[]  SumNumOutMax=[]  DivideOutMin=[]  DivideOutMax=[]  UdiffTsProdOutMin=[]  UdiffTsProdOutMax=[]  NTsProdOutMin=[]  NTsProdOutMax=[]  UintegralTsProdOutMin=[]  UintegralTsProdOutMax=[]  UngainTsProdOutMin=[]  UngainTsProdOutMax=[]  ClampingZeroOutDataTypeStr=Inherit: Inherit via back propagation  ClampingZeroOutMin=[]  ClampingZeroOutMax=[]  FilterDenConstantOutDataTypeStr=Inherit: Inherit via back propagation  FilterDenConstantOutMin=[]  FilterDenConstantOutMax=[]  PCopyOutDataTypeStr=Inherit: Inherit via back propagation  PCopyOutMin=[]  PCopyOutMax=[]  NCopyOutDataTypeStr=Inherit: Inherit via back propagation  NCopyOutMin=[]  NCopyOutMax=[]  IntegratorContinuousStateAttributes=''  IntegratorStateMustResolveToSignalObject=off  IntegratorRTWStateStorageClass=Auto  FilterContinuousStateAttributes=''  FilterStateMustResolveToSignalObject=off  FilterRTWStateStorageClass=Auto  ParallelPVariant=InternalParameters  IdealPVariant=Disabled  IVariant=InternalParameters  DVariant=Disabled  IntegratorVariant=Discrete  SatVariant=Enabled  AWVariant=Passthrough  PCopyVariant=Disabled  TRVariant=Disabled  FdbkBlocksVariant=Forward  IdealPFdbkVariant=Disabled  SatFdbkVariant=Disabled  DerivativeFilterVariant=Disabled  NVariant=Disabled  NCopyVariant=Disabled_SignalSpec  FilterICVariant=Disabled  IntegratorICVariant=InternalICs  ExternalResetVariant=Disabled  TRSumVariant=Passthrough  SumFdbkVariant=Disabled  SumVariant=Sum_PI  TsampFilterVariant=InternalTs  TsampNgainVariant=Passthrough  TsampIntegralVariant=Disabled_SignalSpec  ExternalSaturationOutDataTypeStr=Inherit: Same as second input  DerivativeSourceVariant=Disabled  PreIntVariant=InternalPreInt
  voltage controlled : slpidlib/PID Controller  Controller=PI  Form=Parallel  TimeDomain=Discrete-time  UseExternalTs=off  SampleTime=500e-6  IntegratorMethod=Forward Euler  FilterMethod=Forward Euler  ControllerParametersSource=internal  P=40  I=2000  UseKiTs=off  D=0  UseExternalDerivativeSource=off  N=100  UseFilter=on  TunerSelectOption=Transfer Function Based (PID Tuner App)  InitialConditionSource=internal  InitialConditionForIntegrator=0  InitialConditionForFilter=0  DifferentiatorICPrevScaledInput=0  ExternalReset=none  TrackingMode=off  Kt=1  LimitOutput=on  SatLimitsSource=internal  UpperSaturationLimit=22  LowerSaturationLimit=0  LinearizeAsGain=on  AntiWindupMode=none  Kb=1  LimitIntegrator=off  UpperIntegratorSaturationLimit=inf  LowerIntegratorSaturationLimit=-inf  POutMin=[]  POutMax=[]  IOutMin=[]  IOutMax=[]  DOutMin=[]  DOutMax=[]  NOutMin=[]  NOutMax=[]  SumOutMin=[]  SumOutMax=[]  SaturationOutMin=[]  SaturationOutMax=[]  PParamMin=[]  PParamMax=[]  IParamMin=[]  IParamMax=[]  DParamMin=[]  DParamMax=[]  NParamMin=[]  NParamMax=[]  KbParamMin=[]  KbParamMax=[]  KtParamMin=[]  KtParamMax=[]  KbOutMin=[]  KbOutMax=[]  KtOutMin=[]  KtOutMax=[]  IntegratorOutMin=[]  IntegratorOutMax=[]  FilterOutMin=[]  FilterOutMax=[]  SumI1OutMin=[]  SumI1OutMax=[]  SumI2OutMin=[]  SumI2OutMax=[]  SumI3OutMin=[]  SumI3OutMax=[]  SumI4OutMin=[]  SumI4OutMax=[]  SumDOutMin=[]  SumDOutMax=[]  DifferentiatorOutMin=[]  DifferentiatorOutMax=[]  FilterDiffOutCoefMin=[]  FilterDiffOutCoefMax=[]  ReciprocalOutMin=[]  ReciprocalOutMax=[]  SumDenOutMin=[]  SumDenOutMax=[]  SumNumOutMin=[]  SumNumOutMax=[]  DivideOutMin=[]  DivideOutMax=[]  UdiffTsProdOutMin=[]  UdiffTsProdOutMax=[]  NTsProdOutMin=[]  NTsProdOutMax=[]  UintegralTsProdOutMin=[]  UintegralTsProdOutMax=[]  UngainTsProdOutMin=[]  UngainTsProdOutMax=[]  ClampingZeroOutDataTypeStr=Inherit: Inherit via back propagation  ClampingZeroOutMin=[]  ClampingZeroOutMax=[]  FilterDenConstantOutDataTypeStr=Inherit: Inherit via back propagation  FilterDenConstantOutMin=[]  FilterDenConstantOutMax=[]  PCopyOutDataTypeStr=Inherit: Inherit via back propagation  PCopyOutMin=[]  PCopyOutMax=[]  NCopyOutDataTypeStr=Inherit: Inherit via back propagation  NCopyOutMin=[]  NCopyOutMax=[]  IntegratorContinuousStateAttributes=''  IntegratorStateMustResolveToSignalObject=off  IntegratorRTWStateStorageClass=Auto  FilterContinuousStateAttributes=''  FilterStateMustResolveToSignalObject=off  FilterRTWStateStorageClass=Auto  ParallelPVariant=InternalParameters  IdealPVariant=Disabled  IVariant=InternalParameters  DVariant=Disabled  IntegratorVariant=Discrete  SatVariant=Enabled  AWVariant=Passthrough  PCopyVariant=Disabled  TRVariant=Disabled  FdbkBlocksVariant=Forward  IdealPFdbkVariant=Disabled  SatFdbkVariant=Disabled  DerivativeFilterVariant=Disabled  NVariant=Disabled  NCopyVariant=Disabled_SignalSpec  FilterICVariant=Disabled  IntegratorICVariant=InternalICs  ExternalResetVariant=Disabled  TRSumVariant=Passthrough  SumFdbkVariant=Disabled  SumVariant=Sum_PI  TsampFilterVariant=InternalTs  TsampNgainVariant=Passthrough  TsampIntegralVariant=Disabled_SignalSpec  ExternalSaturationOutDataTypeStr=Inherit: Same as second input  DerivativeSourceVariant=Disabled  PreIntVariant=InternalPreInt
  tag scope: S_N=global, S_P=global
  wires:
  PWM Generator (DC-DC)1/1 -> NOT3/1, [S_P]
  voltage controlled/1 -> Gain1/1
  Constant2/1 -> Add3/1
  Add1/1 -> discharge controlled/1
  [Ib_ref_dis] -> Switch1/3
  Add2/1 -> Current controller/1
  [Ib_ref_charge] -> Switch1/1
  Add3/1 -> voltage controlled/1
  Switch1/1 -> Display4/1, [Ib_ref]
  [Ib_ref] -> Add2/2
  [Vb] -> Add3/2
  Gain1/1 -> Display3/1, [Ib_ref_charge]
  NOT3/1 -> [S_N]
  Constant1/1 -> Add1/1
  discharge controlled/1 -> Display2/1, [Ib_ref_dis]
  Current controller/1 -> PWM Generator (DC-DC)1/1
  [Ib] -> Add2/1
  [Vload] -> Add1/2
  [Control] -> NOT1/1
  NOT1/1 -> Switch1/2

== matlab function SRM_IOT/MPPT and PV Controller/Swapping battery controller/MATLAB Function9 ==
  settings: updateMethod=DISCRETE
  data: SOC input; LoadOn output; ChargingOn output
function [LoadOn, ChargingOn] = chargeDischargeNode(SOC)
    % This function determines the charging and discharging states
    % based on the state of charge (SOC) of the battery.
    % Inputs:
    %   SOC - Current state of charge (0 to 100)
    % Outputs:
    %   LoadOn - Indicator if the load is on (1) or off (0)
    %   ChargingOn - Indicator if charging is active (1) or not (0)

    % Initialize persistent variables to retain state across function calls
    persistent LoadOnPersistent;
    persistent ChargingOnPersistent;

    if isempty(LoadOnPersistent)  % Initialize on first call
        LoadOnPersistent = 1;     % Load is initially on
        ChargingOnPersistent = 0;  % Charging is initially off
    end

    % Logic for charging and discharging based on SOC levels
    if SOC > 80
        LoadOnPersistent = 1;      % Turn load on if SOC is above 80%
        ChargingOnPersistent = 0;   % Turn charging off
    elseif SOC < 40
        LoadOnPersistent = 0;      % Turn load off if SOC is below 40%
        ChargingOnPersistent = 1;   % Start charging
    end

    % Assign output values from persistent variables
    LoadOn = LoadOnPersistent;
    ChargingOn = ChargingOnPersistent;
end

== matlab function SRM_IOT/MPPT and PV Controller/Swapping battery controller/MATLAB Function10 ==
  settings: updateMethod=DISCRETE
  data: SOC input; LoadOn output; ChargingOn output
function [LoadOn, ChargingOn] = chargeDischargeNode(SOC)
    % This function determines the charging and discharging states
    % based on the state of charge (SOC) of the battery.
    % Inputs:
    %   SOC - Current state of charge (0 to 100)
    % Outputs:
    %   LoadOn - Indicator if the load is on (1) or off (0)
    %   ChargingOn - Indicator if charging is active (1) or not (0)

    % Initialize persistent variables to retain state across function calls
    persistent LoadOnPersistent;
    persistent ChargingOnPersistent;

    if isempty(LoadOnPersistent)  % Initialize on first call
        LoadOnPersistent = 1;     % Load is initially on
        ChargingOnPersistent = 0;  % Charging is initially off
    end

    % Logic for charging and discharging based on SOC levels
    if SOC > 80
        LoadOnPersistent = 1;      % Turn load on if SOC is above 80%
        ChargingOnPersistent = 0;   % Turn charging off
    elseif SOC < 40
        LoadOnPersistent = 0;      % Turn load off if SOC is below 40%
        ChargingOnPersistent = 1;   % Start charging
    end

    % Assign output values from persistent variables
    LoadOn = LoadOnPersistent;
    ChargingOn = ChargingOnPersistent;
end

== matlab function SRM_IOT/MPPT and PV Controller/Swapping battery controller/MATLAB Function11 ==
  settings: updateMethod=DISCRETE
  data: SOC input; LoadOn output; ChargingOn output
function [LoadOn, ChargingOn] = chargeDischargeNode(SOC)
    % This function determines the charging and discharging states
    % based on the state of charge (SOC) of the battery.
    % Inputs:
    %   SOC - Current state of charge (0 to 100)
    % Outputs:
    %   LoadOn - Indicator if the load is on (1) or off (0)
    %   ChargingOn - Indicator if charging is active (1) or not (0)

    % Initialize persistent variables to retain state across function calls
    persistent LoadOnPersistent;
    persistent ChargingOnPersistent;

    if isempty(LoadOnPersistent)  % Initialize on first call
        LoadOnPersistent = 1;     % Load is initially on
        ChargingOnPersistent = 0;  % Charging is initially off
    end

    % Logic for charging and discharging based on SOC levels
    if SOC > 80
        LoadOnPersistent = 1;      % Turn load on if SOC is above 80%
        ChargingOnPersistent = 0;   % Turn charging off
    elseif SOC < 40
        LoadOnPersistent = 0;      % Turn load off if SOC is below 40%
        ChargingOnPersistent = 1;   % Start charging
    end

    % Assign output values from persistent variables
    LoadOn = LoadOnPersistent;
    ChargingOn = ChargingOnPersistent;
end

== matlab function SRM_IOT/MPPT and PV Controller/Swapping battery controller/MATLAB Function12 ==
  settings: updateMethod=DISCRETE
  data: SOC input; LoadOn output; ChargingOn output
function [LoadOn, ChargingOn] = chargeDischargeNode(SOC)
    % This function determines the charging and discharging states
    % based on the state of charge (SOC) of the battery.
    % Inputs:
    %   SOC - Current state of charge (0 to 100)
    % Outputs:
    %   LoadOn - Indicator if the load is on (1) or off (0)
    %   ChargingOn - Indicator if charging is active (1) or not (0)

    % Initialize persistent variables to retain state across function calls
    persistent LoadOnPersistent;
    persistent ChargingOnPersistent;

    if isempty(LoadOnPersistent)  % Initialize on first call
        LoadOnPersistent = 1;     % Load is initially on
        ChargingOnPersistent = 0;  % Charging is initially off
    end

    % Logic for charging and discharging based on SOC levels
    if SOC > 80
        LoadOnPersistent = 1;      % Turn load on if SOC is above 80%
        ChargingOnPersistent = 0;   % Turn charging off
    elseif SOC < 40
        LoadOnPersistent = 0;      % Turn load off if SOC is below 40%
        ChargingOnPersistent = 1;   % Start charging
    end

    % Assign output values from persistent variables
    LoadOn = LoadOnPersistent;
    ChargingOn = ChargingOnPersistent;
end
